simulink model "Part4_2_2"  (R2021a)
settings: Solver=VariableStepAuto  StartTime=0.0  StopTime=20  RelTol=1e-3
settings Model: Creator=theod  LastModifiedBy=theod

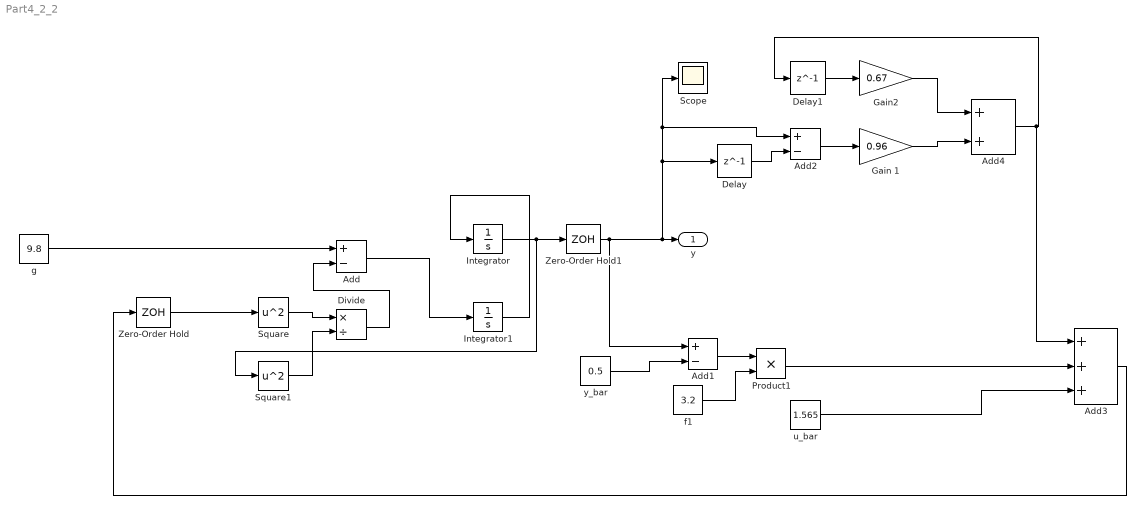
== system Part4_2_2 ==
  Add : Sum  Inputs=+-
  Add1 : Sum  Inputs=+-
  Add2 : Sum  Inputs=+-
  Add3 : Sum  Inputs=+++
  Add4 : Sum
  Delay : Delay  DelayLength=1  InitialCondition=0
  Delay1 : Delay  DelayLength=1  InitialCondition=0
  Divide : Product  Inputs=*/
  Gain 1 : Gain  Gain=0.96
  Gain2 : Gain  Gain=0.67
  Integrator : Integrator  InitialCondition=1.3
  Integrator1 : Integrator  InitialCondition=0.5
  Product1 : Product
  Scope : Scope
  Square : Math  Operator=square  SaturateOnIntegerOverflow=on
  Square1 : Math  Operator=square  SaturateOnIntegerOverflow=on
  Zero-Order Hold : ZeroOrderHold  SampleTime=-1
  Zero-Order Hold1 : ZeroOrderHold  SampleTime=0.05
  f1 : Constant  Value=3.2
  g : Constant  Value=9.8
  u_bar : Constant  Value=1.565
  y_bar : Constant  Value=0.5
  y : Outport
  wires:
  Integrator1/1 -> Integrator/1
  Integrator/1 -> Square1/1, Zero-Order Hold1/1
  Square/1 -> Divide/1
  Square1/1 -> Divide/2
  Divide/1 -> Add/2
  g/1 -> Add/1
  Add/1 -> Integrator1/1
  y_bar/1 -> Add1/2
  Add1/1 -> Product1/1
  f1/1 -> Product1/2
  Product1/1 -> Add3/2
  u_bar/1 -> Add3/3
  Zero-Order Hold/1 -> Square/1
  Add3/1 -> Zero-Order Hold/1
  Zero-Order Hold1/1 -> Delay/1, Add2/1, Scope/1, y/1, Add1/1
  Delay/1 -> Add2/2
  Add2/1 -> Gain 1/1
  Gain 1/1 -> Add4/2
  Add4/1 -> Add3/1, Delay1/1
  Delay1/1 -> Gain2/1
  Gain2/1 -> Add4/1
